simulink model "Qn4"  (R2022b)
settings: Solver=VariableStepAuto  StartTime=0.0  StopTime=10.0  RelTol=1e-3
settings Model: Creator=nmary  LastModifiedBy=nmary

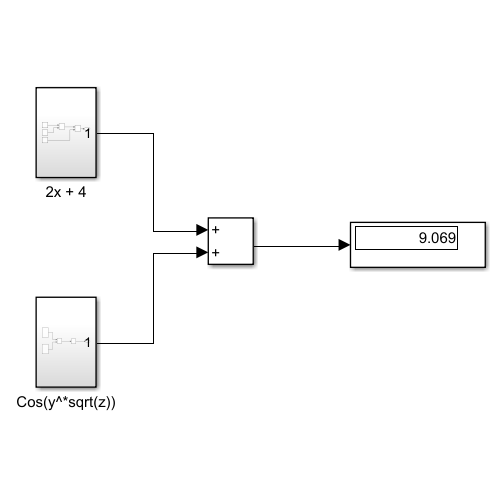
[thumbnail: Simulink's stored preview of the top-level diagram]
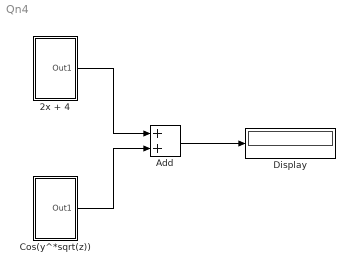
== system Qn4 ==
  2x + 4 : Subsystem
  Add : Sum
  Cos(y^*sqrt(z)) : Subsystem
  Display : Display
  wires:
  2x + 4/1(Out1) -> Add/1
  Cos(y^*sqrt(z))/1(Out1) -> Add/2
  Add/1 -> Display/1

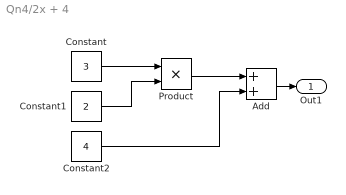
== system Qn4/2x + 4 ==
  Add : Sum
  Constant : Constant  Value=3
  Constant1 : Constant  Value=2
  Constant2 : Constant  Value=4
  Product : Product
  Out1 : Outport
  wires:
  Add/1 -> Out1/1
  Product/1 -> Add/1
  Constant1/1 -> Product/2
  Constant/1 -> Product/1
  Constant2/1 -> Add/2

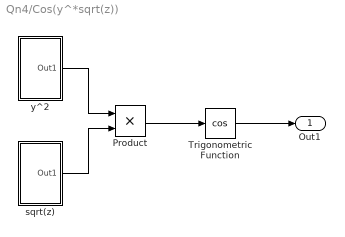
== system Qn4/Cos(y^*sqrt(z)) ==
  Product : Product
  Trigonometric Function : Trigonometry  Operator=cos
  sqrt(z) : Subsystem
  y^2 : Subsystem
  Out1 : Outport
  wires:
  y^2/1(Out1) -> Product/1
  Product/1 -> Trigonometric Function/1
  sqrt(z)/1(Out1) -> Product/2
  Trigonometric Function/1 -> Out1/1

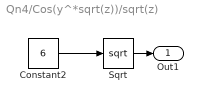
== system Qn4/Cos(y^*sqrt(z))/sqrt(z) ==
  Constant2 : Constant  Value=6
  Sqrt : Sqrt
  Out1 : Outport
  wires:
  Constant2/1 -> Sqrt/1
  Sqrt/1 -> Out1/1

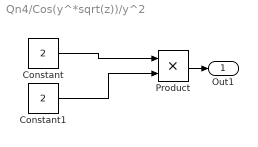
== system Qn4/Cos(y^*sqrt(z))/y^2 ==
  Constant : Constant  Value=2
  Constant1 : Constant  Value=2
  Product : Product
  Out1 : Outport
  wires:
  Constant1/1 -> Product/2
  Constant/1 -> Product/1
  Product/1 -> Out1/1
